simulink model "modPSK"  (R2022a)
settings: Solver=VariableStepAuto  StartTime=0.0  StopTime=1500*Tb
values from neighbouring files (symbols this model uses):
  Amplitud = 1    [SincronizmoPSK.m]    (also in calculoVariablesTransmisionPSK.m)
  AmplitudPortadora = 2.326*sqrt(eta/Tb)    [SincronizmoPSK.m]    (also in calculoVariablesTransmisionPSK.m)
  Ancho_banda_minimo = Rb / 2    (= 5000)    [SincronizmoPSK.m]    (also in calculoVariablesTransmisionPSK.m)
  AnchoDeBandaRuido = 2E6    (= 2000000)    [SincronizmoPSK.m]    (also in calculoVariablesTransmisionPSK.m)
  Att_pot_Canal = 10^(Att_dB / 10)    [SincronizmoPSK.m]    (also in calculoVariablesTransmisionPSK.m)
  Att_Volt_Canal = 10^(Att_dB / 20)    [SincronizmoPSK.m]    (also in calculoVariablesTransmisionPSK.m)
  b = 0.85    [SincronizmoPSK.m]    (also in calculoVariablesTransmisionPSK.m)
  C = 1e-6    (= 1e-06)    [SincronizmoPSK.m]    (also in calculoVariablesTransmisionPSK.m)
  Frec_port = 1e6    (= 1000000)    [SincronizmoPSK.m]    (also in calculoVariablesTransmisionPSK.m)
  Kv = 1E5    (= 100000)    [SincronizmoPSK.m]    (also in calculoVariablesTransmisionPSK.m)
  Pot_Ruido = Pot_Ruido/2    (= 2.0709e-15)    [SincronizmoPSK.m]    (also in calculoVariablesTransmisionPSK.m = 4.1418e-15)
  R1 = Kp * Kv / (wn^2 * C)    (= 0.987654320988)    [SincronizmoPSK.m]    (also in calculoVariablesTransmisionPSK.m)
  R2 = 2 * zita / (wn * C)    (= 5.33333333333)    [SincronizmoPSK.m]    (also in calculoVariablesTransmisionPSK.m)
  Rb = 1e4    (= 10000)    [SincronizmoPSK.m]    (also in calculoVariablesTransmisionPSK.m)
  Retraso_Canal = Long_Canal / C_canal+0.5/Frec_port    (= 0.0010005)    [SincronizmoPSK.m]    (also in calculoVariablesTransmisionPSK.m)
  Tb = 1 / Rb    (= 0.0001)    [SincronizmoPSK.m]    (also in calculoVariablesTransmisionPSK.m)
libraries: dsparch4 x4, dspsigops x3, commsynccomp2 x2, powerlib_extras x2, dspsnks4 x2, spsMonostableLib x1, simulink_extras x1, dspsrcs4 x1
settings Model: SimulationMode=accelerator  SILPILSystemUnderTest=refmodels  SILPILSimulationModeTopModel=rapid-accelerator  SILPILSimulationModeModelRef=accelerator  Creator=Daniel  LastModifiedBy=Juan Carlos
settings SolverCC: ZeroCrossControl=DisableAll  ZeroCrossAlgorithm=Adaptive  InsertRTBMode=Never (minimum delay)
settings OptimizationCC: InitFltsAndDblsToZero=on
settings DebuggingCC: UnconnectedInputMsg=warning  UnconnectedOutputMsg=warning  UnconnectedLineMsg=warning
settings HardwareCC: ProdHWDeviceType=AMD->x86-64 (Windows64)  TargetLongLongMode=on
settings ModelReferenceCC: EnableParallelModelReferenceBuilds=on  ParallelModelReferenceMATLABWorkerInit=Copy Base Workspace
settings SFSimCC: SimTargetLang=C++  SimGPUCustomComputeCapability=6.1
settings RTWCC: Toolchain=MinGW64 | gmake (64-bit Windows)  GPUDeviceID=1  GPUEnableMemoryManager=on  GPUComputeCapability=6.1  GPUMaximumBlocksPerKernel=64  DLArmComputeVersion=19.05

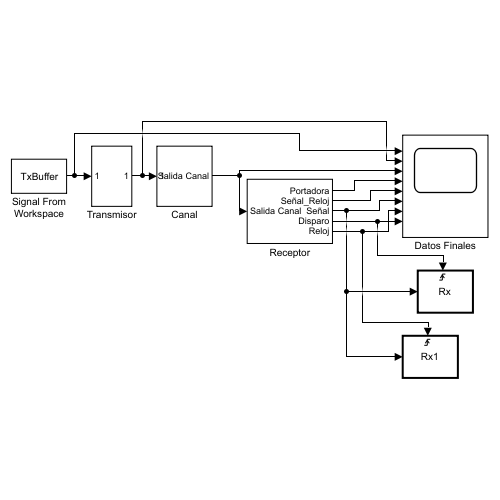
[thumbnail: Simulink's stored preview of the top-level diagram]
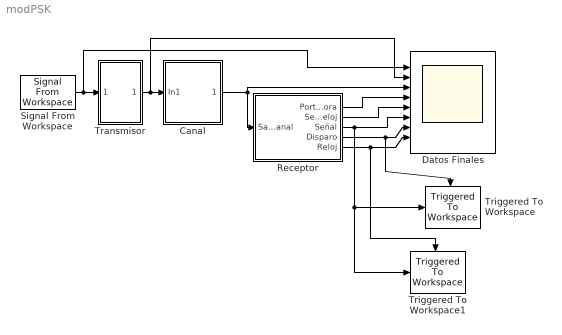
== system modPSK ==
  Canal : Subsystem
  Datos Finales : Scope  NumInputPorts=8
  Receptor : Subsystem
  Signal From Workspace : dspsrcs4/Signal From Workspace  X=TxBuffer  Ts=Tb  nsamps=1  OutputAfterFinalValue=Setting to zero  ignoreOrWarnInputAndFrameLengths=off  OutputFrames=off
  Transmisor : Subsystem
  Triggered To Workspace : dspsnks4/Triggered To Workspace  TriggerType=Rising edge  VariableName=Rx  Buffer=2000  Save2DMode=2-D array (concatenate along first dimension)
      settings: SourceProductBaseCode=DS  FixptAsFi=off
  Triggered To Workspace1 : dspsnks4/Triggered To Workspace  TriggerType=Rising edge  VariableName=Rx1  Buffer=2000  Save2DMode=2-D array (concatenate along first dimension)
      settings: SourceProductBaseCode=DS  FixptAsFi=off
  wires:
  Signal From Workspace/1 -> Datos Finales/1, Transmisor/1(In2)
  Transmisor/1(Out1) -> Datos Finales/2, Canal/1(In1)
  Canal/1(Salida Canal) -> Receptor/1(Salida Canal), Datos Finales/3
  Receptor/1(Portadora) -> Datos Finales/4
  Receptor/2(Señal_Reloj) -> Datos Finales/5
  Receptor/3(Señal) -> Triggered To Workspace1/1, Triggered To Workspace/1, Datos Finales/6
  Receptor/4(Disparo) -> Triggered To Workspace/Trigger, Datos Finales/7
  Receptor/5(Reloj) -> Triggered To Workspace1/Trigger, Datos Finales/8

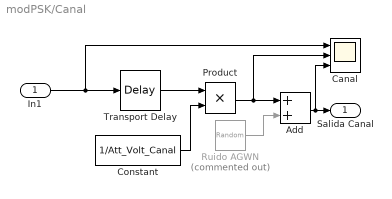
== system modPSK/Canal ==
  In1 : Inport
  Add : Sum
  Canal : Scope  NumInputPorts=3
  Constant : Constant  Value=1/Att_Volt_Canal
  Product : Product
  Ruido AGWN : RandomNumber  Commented=on  Variance=Pot_Ruido  SampleTime=1/(2*AnchoDeBandaRuido)
  Transport Delay : TransportDelay  DelayTime=Retraso_Canal  BufferSize=1024*10
  Salida Canal : Outport
  wires:
  Constant/1 -> Product/2
  Product/1 -> Canal/2, Add/1
  Ruido AGWN/1 -> Add/2
  Add/1 -> Canal/3, Salida Canal/1
  Transport Delay/1 -> Product/1
  In1/1 -> Canal/1, Transport Delay/1

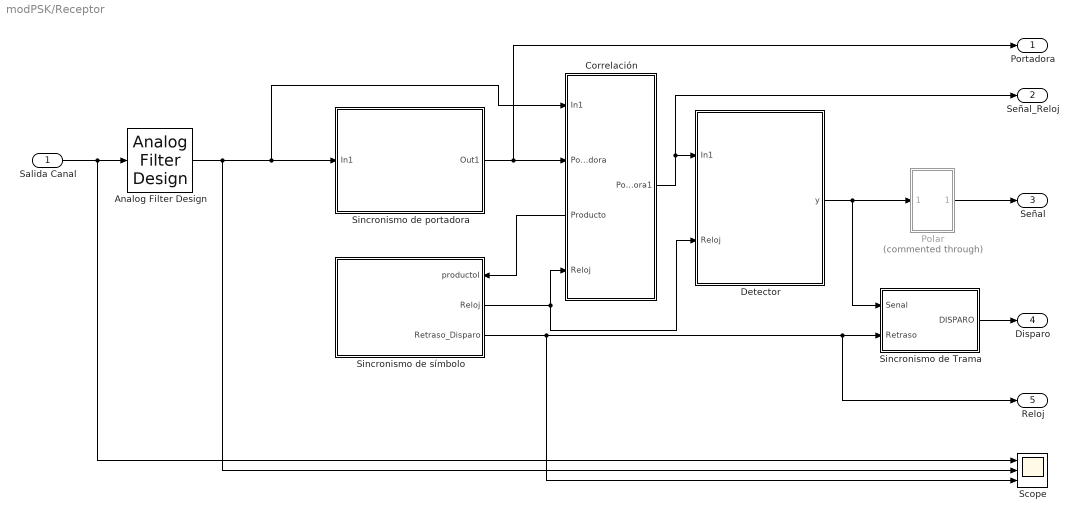
== system modPSK/Receptor ==
  Salida Canal : Inport
  Analog Filter Design : dsparch4/Analog Filter Design  method=Butterworth  filttype=Bandpass  N=2  Wlo=2*pi*(Frec_port - 2*Ancho_banda_minimo)  Whi=2*pi*(Frec_port + 2*Ancho_banda_minimo)  Rp=2  Rs=40
  Correlación : Subsystem
      settings: PortSchema="{\"entries\":[{\"content\":{\"sides\":[{\"content\":{\"connectorIds\":[\"In1\",\"In2\",\"Out2\",\"In3\"]},\"type\":\"ConnectorPlacement.EquallySpacedRectSide\",\"uuid\":\"9c9ed9ca-e8ca-44c2-a659-85a067b2e2ab\"},{\"content\":{\"connectorIds\":[\"Out1\"],\"side\":\"RIGHT\"},\"type\":\"ConnectorPlacement.EquallySpacedRectSide\",\"uuid\":\"749548a8-d339-4a18-8c47-3529cad88115\"},{\"content\":{\"connectorIds\":[],\"side\":\"TOP\"},\"type\":\"ConnectorPlacement.EquallySpacedRectSide\",\"uuid\":\"502cb8ca-7e6c-4f6d-9acf-9edc021ca5d9\"},{\"content\":{\"connectorIds\":[],\"side\":\"BOTTOM\"},\"type\":\"ConnectorPlacement.EquallySpacedRectSide\",\"uuid\":\"343f95ab-8b43-4ca2-96bf-a55a52c277fe\"}]},\"type\":\"ConnectorPlacement.EquallySpacedConnector\",\"uuid\":\"c50381c4-8798-4039-a023-6424d6fa731c\"}],\"packageUris\":[\"http://schema.mathworks.com/mf0/Connector/R2020b\"],\"version\":\"1.0\"}"
  Detector : Subsystem
  Polar : Subsystem  Commented=through
  Scope : Scope  NumInputPorts=3
  Sincronismo de Trama : Subsystem
  Sincronismo de portadora : Subsystem
  Sincronismo de símbolo : Subsystem
      settings: PortSchema="{\"entries\":[{\"content\":{\"sides\":[{\"content\":{\"connectorIds\":[]},\"type\":\"ConnectorPlacement.EquallySpacedRectSide\",\"uuid\":\"93994b0c-b2cb-4331-9695-4cda4bbb6019\"},{\"content\":{\"connectorIds\":[\"In1\",\"Out1\",\"Out2\"],\"side\":\"RIGHT\"},\"type\":\"ConnectorPlacement.EquallySpacedRectSide\",\"uuid\":\"b8064540-0ede-4985-840d-1e59709fa35b\"},{\"content\":{\"connectorIds\":[],\"side\":\"TOP\"},\"type\":\"ConnectorPlacement.EquallySpacedRectSide\",\"uuid\":\"0f7e7988-f1a5-40c2-b0ce-e0a51a477c0a\"}]},\"type\":\"ConnectorPlacement.EquallySpacedConnector\",\"uuid\":\"3553a0bb-71d1-453e-9ff3-b6164d2735c0\"}],\"packageUris\":[\"http://schema.mathworks.com/mf0/Connector/R2020b\"],\"version\":\"1.0\"}"
  Portadora : Outport
  Señal_Reloj : Outport  Port=2
  Señal : Outport  Port=3
  Disparo : Outport  Port=4
  Reloj : Outport  Port=5
  wires:
  Correlación/1(Portadora1) -> Señal_Reloj/1, Detector/1(In1)
  Detector/1(y) -> Sincronismo de Trama/1(Senal), Polar/1(In1)
  Sincronismo de portadora/1(Out1) -> Portadora/1, Correlación/2(Portadora)
  Sincronismo de símbolo/1(Reloj) -> Detector/2(Reloj), Correlación/3(Reloj)
  Correlación/2(Producto) -> Sincronismo de símbolo/1(productol)
  Polar/1(Out1) -> Señal/1
  Sincronismo de Trama/1("DISPARO ") -> Disparo/1
  Salida Canal/1 -> Scope/1, Analog Filter Design/1
  Analog Filter Design/1 -> Scope/2, Correlación/1(In1), Sincronismo de portadora/1(In1)
  Sincronismo de símbolo/2(Retraso_Disparo) -> Scope/3, Reloj/1, Sincronismo de Trama/2(Retraso)

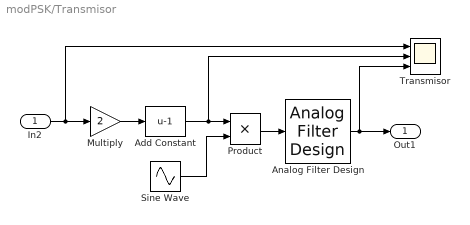
== system modPSK/Transmisor ==
  In2 : Inport
  Add Constant : Bias  Bias=-1  SaturateOnIntegerOverflow=off
  Analog Filter Design : dsparch4/Analog Filter Design  method=Butterworth  filttype=Bandpass  N=2  Wlo=2*pi*(Frec_port - 2 *Ancho_banda_minimo)  Whi=2*pi*(Frec_port + 2 *Ancho_banda_minimo)  Rp=2  Rs=40
  Multiply : Gain  Gain=2
  Product : Product
  Sine Wave : Sin  Amplitude=AmplitudPortadora  Frequency=2*pi*Frec_port  Samples=5  SampleTime=0
  Transmisor : Scope  NumInputPorts=3
  Out1 : Outport
  wires:
  Multiply/1 -> Add Constant/1
  Add Constant/1 -> Transmisor/2, Product/1
  Analog Filter Design/1 -> Transmisor/3, Out1/1
  In2/1 -> Transmisor/1, Multiply/1
  Product/1 -> Analog Filter Design/1
  Sine Wave/1 -> Product/2

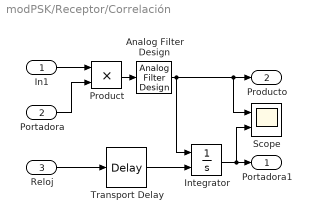
== system modPSK/Receptor/Correlación ==
  In1 : Inport
  Portadora : Inport  Port=2
  Reloj : Inport  Port=3
  Analog Filter Design : dsparch4/Analog Filter Design  method=Butterworth  filttype=Lowpass  N=8  Wlo=2*pi*Rb  Whi=80  Rp=2  Rs=40
  Integrator : Integrator  ExternalReset=rising
  Product : Product
  Scope : Scope  NumInputPorts=2
  Transport Delay : TransportDelay  DelayTime=1e-9
  Portadora1 : Outport
  Producto : Outport  Port=2
  wires:
  Transport Delay/1 -> Integrator/2
  In1/1 -> Product/1
  Integrator/1 -> Scope/2, Portadora1/1
  Reloj/1 -> Transport Delay/1
  Product/1 -> Analog Filter Design/1
  Portadora/1 -> Product/2
  Analog Filter Design/1 -> Integrator/1, Scope/1, Producto/1

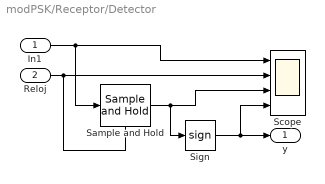
== system modPSK/Receptor/Detector ==
  In1 : Inport
  Reloj : Inport  Port=2
  Sample and Hold : dspsigops/Sample and Hold  trig=Rising edge  initCond=0  latchinput=off
  Scope : Scope  NumInputPorts=4
  Sign : Signum
  y : Outport
  wires:
  In1/1 -> Scope/1, Sample and Hold/1
  Sign/1 -> Scope/4, y/1
  Sample and Hold/1 -> Scope/3, Sign/1
  Reloj/1 -> Scope/2, Sample and Hold/Trigger

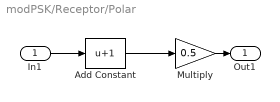
== system modPSK/Receptor/Polar ==
  In1 : Inport
  Add Constant : Bias  Bias=1  SaturateOnIntegerOverflow=off
  Multiply : Gain  Gain=0.5
  Out1 : Outport
  wires:
  Add Constant/1 -> Multiply/1
  Multiply/1 -> Out1/1
  In1/1 -> Add Constant/1

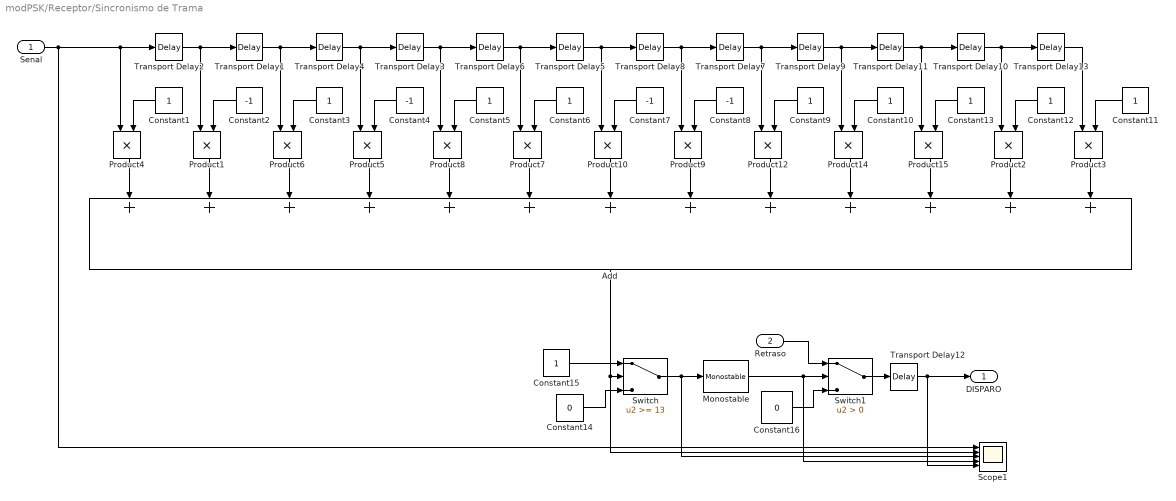
== system modPSK/Receptor/Sincronismo de Trama ==
  Senal : Inport
  Retraso : Inport  Port=2
  Add : Sum  Inputs=+++++++++++++
  Constant{1,3,5..6,9..13,15} (10 alike) : Constant
  Constant14 : Constant  Value=0
  Constant16 : Constant  Value=0
  Constant{2,4,7..8} (4 alike) : Constant  Value=-1
  Monostable : spsMonostableLib/Monostable  EdgeDetect=Rising  PulseDuration=1000*Tb  ic=0  Ts=0
      settings: SourceProductBaseCode=PS
  Product{1..10,12,14..15} (13 alike) : Product
  Scope1 : Scope  NumInputPorts=5
  Switch : Switch  Threshold=13  SaturateOnIntegerOverflow=off  InputSameDT=off
  Switch1 : Switch  Criteria=u2 > Threshold  SaturateOnIntegerOverflow=off  InputSameDT=off
  Transport Delay{1..11,13} (12 alike) : TransportDelay  DelayTime=Tb
  Transport Delay12 : TransportDelay  DelayTime=Tb/50
  "DISPARO " : Outport  VectorParamsAs1DForOutWhenUnconnected=off
  wires:
  Transport Delay6/1 -> Product7/1, Transport Delay5/1
  Constant7/1 -> Product10/2
  Monostable/1 -> Scope1/4, Switch1/2
  Constant1/1 -> Product4/2
  Transport Delay1/1 -> Product6/1, Transport Delay4/1
  Product7/1 -> Add/6
  Transport Delay4/1 -> Product5/1, Transport Delay3/1
  Transport Delay3/1 -> Product8/1, Transport Delay6/1
  Constant13/1 -> Product15/2
  Transport Delay12/1 -> Scope1/5, "DISPARO "/1
  Add/1 -> Scope1/2, Switch/2
  Product4/1 -> Add/1
  Product14/1 -> Add/10
  Constant6/1 -> Product7/2
  Product6/1 -> Add/3
  Product9/1 -> Add/8
  Product5/1 -> Add/4
  Senal/1 -> Product4/1, Transport Delay2/1, Scope1/1
  Constant5/1 -> Product8/2
  Transport Delay5/1 -> Product10/1, Transport Delay8/1
  Constant16/1 -> Switch1/3
  Constant15/1 -> Switch/1
  Transport Delay9/1 -> Product14/1, Transport Delay11/1
  Constant4/1 -> Product5/2
  Transport Delay8/1 -> Product9/1, Transport Delay7/1
  Product8/1 -> Add/5
  Constant14/1 -> Switch/3
  Constant9/1 -> Product12/2
  Constant3/1 -> Product6/2
  Constant10/1 -> Product14/2
  Product10/1 -> Add/7
  Switch/1 -> Scope1/3, Monostable/1
  Product15/1 -> Add/11
  Transport Delay7/1 -> Product12/1, Transport Delay9/1
  Transport Delay11/1 -> Transport Delay10/1, Product15/1
  Switch1/1 -> Transport Delay12/1
  Constant8/1 -> Product9/2
  Transport Delay2/1 -> Product1/1, Transport Delay1/1
  Constant2/1 -> Product1/2
  Retraso/1 -> Switch1/1
  Product1/1 -> Add/2
  Product12/1 -> Add/9
  Product2/1 -> Add/12
  Product3/1 -> Add/13
  Transport Delay10/1 -> Product2/1, Transport Delay13/1
  Constant11/1 -> Product3/2
  Constant12/1 -> Product2/2
  Transport Delay13/1 -> Product3/1

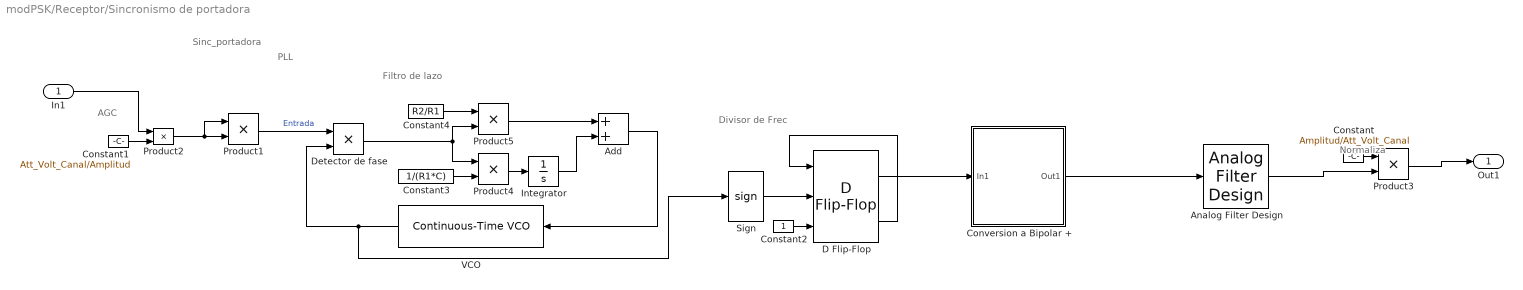
== system modPSK/Receptor/Sincronismo de portadora ==
  note: Filtro de lazo
  note: Divisor de Frec
  note: PLL
  note: Normaliza
  note: Sinc_portadora
  note: AGC
  In1 : Inport
  " VCO" : commsynccomp2/Continuous-Time VCO  Ac=1  Fc=2*Frec_port  Kc=Kv/(2*pi)  Ph=0
      settings: SourceProductBaseCode=CM
  Add : Sum
  Analog Filter Design : dsparch4/Analog Filter Design  method=Butterworth  filttype=Bandpass  N=2  Wlo=1.8*pi*Frec_port  Whi=2.2*pi*Frec_port  Rp=2  Rs=40
  Constant : Constant  Value=Amplitud/Att_Volt_Canal
  Constant1 : Constant  Value=Att_Volt_Canal/Amplitud
  Constant2 : Constant
  Constant3 : Constant  Value=1/(R1*C)
  Constant4 : Constant  Value=R2/R1
  Conversion a Bipolar + : Subsystem
  D Flip-Flop : simulink_extras/Flip Flops/D Flip-Flop
  Detector de fase : Product
  Integrator : Integrator
  Product{1..5} (5 alike) : Product
  Sign : Signum
  Out1 : Outport
  wires:
  Product3/1 -> Out1/1
  In1/1 -> Product2/1
  Constant1/1 -> Product2/2
  Product2/1 -> Product1/1, Product1/2
  Constant/1 -> Product3/1
  Add/1 -> " VCO"/1
  Product1/1 -> Detector de fase/1  "Entrada"
  Sign/1 -> D Flip-Flop/2
  " VCO"/1 -> Detector de fase/2, Sign/1
  D Flip-Flop/2 -> D Flip-Flop/1
  Constant2/1 -> D Flip-Flop/3
  Constant4/1 -> Product5/1
  Product5/1 -> Add/1
  Detector de fase/1 -> Product5/2, Product4/1
  Product4/1 -> Integrator/1
  Integrator/1 -> Add/2
  Constant3/1 -> Product4/2
  Analog Filter Design/1 -> Product3/2
  D Flip-Flop/1 -> Conversion a Bipolar +/1(In1)
  Conversion a Bipolar +/1(Out1) -> Analog Filter Design/1

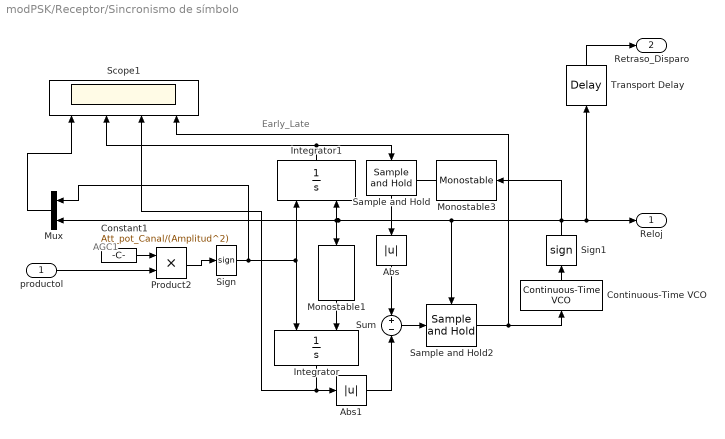
== system modPSK/Receptor/Sincronismo de símbolo ==
  note: Early_Late
  note: AGC1
  productol : Inport
  Abs : Abs  SaturateOnIntegerOverflow=off
  Abs1 : Abs  SaturateOnIntegerOverflow=off
  Constant1 : Constant  Value=Att_pot_Canal/(Amplitud^2)
  Continuous-Time VCO : commsynccomp2/Continuous-Time VCO  Ac=1  Fc=Rb  Kc=kv2  Ph=1.75*pi
      settings: SourceProductBaseCode=CM
  Integrator : Integrator  ExternalReset=falling  UpperSaturationLimit=0.7e-4  LowerSaturationLimit=-0.7e-4
  Integrator1 : Integrator  ExternalReset=rising  UpperSaturationLimit=0.7e-4  LowerSaturationLimit=-0.7e-4
  Monostable1 : powerlib_extras/Control  Blocks/Monostable  EdgeDetect=Rising  t_mono=(1-b)/Rb  ic=0
      settings: SourceProductBaseCode=PS
  Monostable3 : powerlib_extras/Control  Blocks/Monostable  EdgeDetect=Falling  t_mono=b/Rb  ic=0
      settings: SourceProductBaseCode=PS
  Mux : Mux  Inputs=2
  Product2 : Product
  Sample and Hold : dspsigops/Sample and Hold  trig=Rising edge  initCond=0  latchinput=off
  Sample and Hold2 : dspsigops/Sample and Hold  trig=Rising edge  initCond=0  latchinput=off
  Scope1 : Scope  NumInputPorts=4
  Sign : Signum
  Sign1 : Signum
  Sum : Sum  Inputs=+-
  Transport Delay : TransportDelay  DelayTime=Tb/50
  Reloj : Outport
  Retraso_Disparo : Outport  Port=2
  wires:
  Sign1/1 -> Monostable3/1, Monostable1/1, Mux/2, Integrator1/2, Sample and Hold2/Trigger, Transport Delay/1, Reloj/1
  Product2/1 -> Sign/1
  Constant1/1 -> Product2/1
  productol/1 -> Product2/2
  Sign/1 -> Integrator/1, Integrator1/1, Mux/1
  Continuous-Time VCO/1 -> Sign1/1
  Abs/1 -> Sum/1
  Sum/1 -> Sample and Hold2/1
  Integrator1/1 -> Sample and Hold/1, Scope1/2
  Abs1/1 -> Sum/2
  Sample and Hold/1 -> Abs/1
  Integrator/1 -> Scope1/3, Abs1/1
  Monostable3/1 -> Sample and Hold/Trigger
  Monostable1/1 -> Integrator/2
  Sample and Hold2/1 -> Continuous-Time VCO/1, Scope1/4
  Mux/1 -> Scope1/1
  Transport Delay/1 -> Retraso_Disparo/1

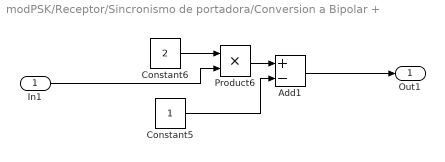
== system modPSK/Receptor/Sincronismo de portadora/Conversion a Bipolar + ==
  In1 : Inport
  Add1 : Sum  Inputs=+-
  Constant5 : Constant
  Constant6 : Constant  Value=2
  Product6 : Product
  Out1 : Outport
  wires:
  Product6/1 -> Add1/1
  Constant5/1 -> Add1/2
  Constant6/1 -> Product6/1
  In1/1 -> Product6/2
  Add1/1 -> Out1/1
